simulink model "SolverLab1"  (R2020a)
settings: Solver=ode45  StartTime=0.0  StopTime=10.0  RelTol=1e-3
settings Model: Creator=Ganesh  LastModifiedBy=Ganesh

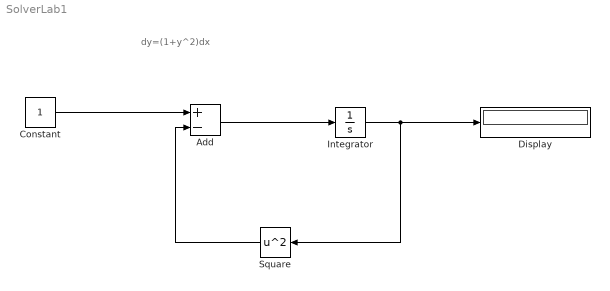
== system SolverLab1 ==
  note: dy=(1+y^2)dx
  Add : Sum  Inputs=+-
  Constant : Constant
  Display : Display
  Integrator : Integrator  InitialCondition=1
  Square : Math  Operator=square  SaturateOnIntegerOverflow=on
  wires:
  Constant/1 -> Add/1
  Add/1 -> Integrator/1
  Integrator/1 -> Display/1, Square/1
  Square/1 -> Add/2
